simulink model "TargetAttitudeGenerator"  (Simulink 7.3)
settings: Solver=ode45  StartTime=0.0  StopTime=10.0  RelTol=1e-3
settings Model: Creator=Owner  LastModifiedBy=Owner

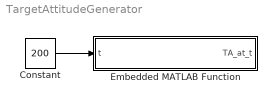
== system TargetAttitudeGenerator ==
  Constant : Constant  Value=200  OutDataType=fixdt(1, 16)  OutScaling=2^0
  Embedded MATLAB Function : Stateflow chart
  wires:
  Constant/1 -> Embedded MATLAB Function/1(t)

== matlab function Embedded MATLAB Function ==
  data: t input double; TA_at_t output double
function TA_at_t  = TargetAttitude(t)

eml.extrinsic('ECIOrbitModel');
eml.extrinsic('DCMECItoECEF');
eml.extrinsic('igrf11syn');
eml.extrinsic('TargetAttitude');
eml.extrinsic('GHcoefficients');

TA_at_t=zeros(3,3);
t_sim=6000; %seconds
time_step=100; %seconds

%orbit parameters
altitude=800000;
Omega=257.65*pi/180; %RAAN
omega=0; %argument of perigee. Has no significance for a circular orbit. 
%If an elliptical orbit is required, modifications must be made to the
%function ECIOrbitModel.
%%%%%%%%%%%%%%%%%%%%%%%%%%%%%%%%%%%%%%%%%%%%%%%%%%%%%%%%%%%%%%%%%%%%%%%%%%

close all
num=t_sim/time_step;
TA=zeros(3,3,num);
oo=1;
    inclination=(100-10*oo)*pi/180;
    dip=zeros(1,num);
    TA=zeros(3,3,num);
    lat=zeros(1,num);
    long=zeros(1,num);
    r_ECEF=zeros(3,num);
    for t=1:num
        r_ECI=ECIOrbitModel(time_step*t,Omega,inclination,omega,altitude);
        r_ECEF(:,t)=DCMECItoECEF(time_step*t)*r_ECI;
        [lat(t) long(t)]=LatLong(r_ECEF(:,t));

        %initializing IGRF
       
        if exist('GHcoefficients','file')==2
            load('GHcoefficients')
        else
            gh=GetIGRF11_Coefficients(1);
        end
        
        %Finding B, dip, and target attitude (here, target attitude assumes
        %the Cones-Not-Intersecting case.)
        B_ECEF_sph=igrf11syn(2011,800,lat(t),long(t));
        dip(t)=atand(-B_ECEF_sph(3)/sqrt(B_ECEF_sph(2)^2+B_ECEF_sph(1)^2));
        TA(:,:,t)=TargetAttitude([B_ECEF_sph(1);B_ECEF_sph(2);-B_ECEF_sph(3)]);
    end
TA_at_t=TA(:,:,t);
